simulink model "crop_simulation"  (R2021a)
settings: Solver=ode23tb  StartTime=0.0  StopTime=4  RelTol=1e-2
values from neighbouring files (symbols this model uses):
  parameters = LoadParameters()    [OnlyPlots.m]    (also in run_crop_simulation.m; run_several_crop_simulation.m)
undefined symbols (not defined in the file or in its folder): climate_GH3, MM_vec, nearst_p, p, PowerArtificial, Tr, Tref, Ts, x0_SOFC
libraries: HORTISIM x14, pid_lib x4
(part 1 of 3)
settings Model: SimulationMode=accelerator  Creator=izaro.garro  LastModifiedBy=djoroya
settings SolverCC: AlgebraicLoopSolver=TrustRegion  MinimalZcImpactIntegration=on
settings DebuggingCC: UnconnectedInputMsg=none  UnconnectedOutputMsg=none  UnconnectedLineMsg=none  SFMachineParentedDataDiag=warning
settings SFSimCC: CustomCodeUndefinedFunction=UseInterfaceOnly

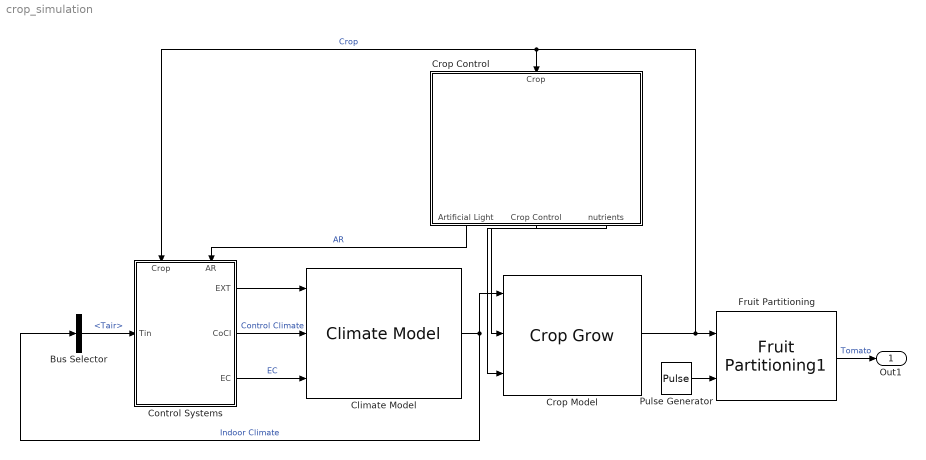
== system crop_simulation ==
  Bus Selector : BusSelector  OutputSignals=Temp.Tair
  Climate Model : HORTISIM/Climate/Models/Climate Model  G0=parameters.climate.G0  T0=parameters.climate.T0  H=parameters.climate.H  A_f=parameters.climate.A_f  A_c=parameters.climate.A_c  minWindows=parameters.climate.minWindows  lam_s=parameters.climate.lam_s  c_s=parameters.climate.c_s  l_s=parameters.climate.l_s  rhod_s=parameters.climate.rhod_s  int_air_speed=parameters.climate.int_air_speed  alpha_i=parameters.climate.alpha_i  alpha_c=parameters.climate.alpha_c  tau_c=parameters.climate.tau_c  alpha_f=parameters.climate.alpha_f  d_c=parameters.climate.d_c  cd_c=parameters.climate.cd_c  T_ss=parameters.climate.T_ss
      settings: SourceProductName=Horti Simulator
  Control Systems : Subsystem
      settings: PortSchema="{\"entries\":[{\"content\":{\"sides\":[{\"content\":{\"connectorIds\":[\"In1\"]},\"type\":\"ConnectorPlacement.EquallySpacedRectSide\",\"uuid\":\"2391a20f-f100-4cab-96a6-b0b26723d027\"},{\"content\":{\"connectorIds\":[\"Out1\",\"Out2\",\"Out3\"],\"side\":\"RIGHT\"},\"type\":\"ConnectorPlacement.EquallySpacedRectSide\",\"uuid\":\"6fe3ba53-dc35-4946-8b7e-8d400e08f612\"},{\"content\":{\"connectorIds\":[\"In2\",\"In3\"],\"side\":\"TOP\"},\"type\":\"ConnectorPlacement.EquallySpacedRectSide\",\"uuid\":\"3c9d9863-f637-4420-aa21-e61bd2fd014c\"}]},\"type\":\"ConnectorPlacement.EquallySpacedConnector\",\"uuid\":\"bf96f136-6ce3-41a6-8557-bc451a3eeee3\"}],\"packageUris\":[\"http://schema.mathworks.com/mf0/Connector/R2020b\"],\"version\":\"1.0\"}"
  Crop Control : Subsystem
  Crop Model : HORTISIM/Horticulture/Models/Crop Grow  Chi_nutrients=parameters.crop.Chi_nutrients  A_v=parameters.crop.A_v  plants_density=parameters.crop.plants_density  fraction_DM=parameters.crop.fraction_DM  min_water_capacity=parameters.crop.min_water_capacity  C_buf_max=parameters.crop.C_buf_max  T_v_start_fruit=parameters.crop.T_v_start_fruit  int_air_speed=parameters.crop.int_air_speed  b_N_uptake=parameters.crop.b_N_uptake  Tv=parameters.crop.Tv  C=parameters.crop.C  R=parameters.crop.R  Tsum=parameters.crop.Tsum  C_wv=parameters.crop.C_wv  N=parameters.crop.N  rg_fruit=parameters.crop.rg_fruit  c_fruit_m=parameters.crop.c_fruit_m  c_fruit_g=parameters.crop.c_fruit_g  rg_leaf=parameters.crop.rg_leaf  c_leaf_m=parameters.crop.c_leaf_m  c_leaf_g=parameters.crop.c_leaf_g  rg_stem=parameters.crop.rg_stem  c_stem_m=parameters.crop.c_stem_m  c_stem_g=parameters.crop.c_stem_g  VelocityAbsortion=parameters.crop.VelocityAbsortion  T_max_v=parameters.crop.T_max_v  s_max_T=parameters.crop.s_max_T  s_min_T=parameters.crop.s_min_T  s_buforg_buf=parameters.crop.s_buforg_buf  T_sum_end=parameters.crop.T_sum_end  T_max_v24=parameters.crop.T_max_v24  T_min_v24=parameters.crop.T_min_v24  s_min_T24=parameters.crop.s_min_T24  s_max_T24=parameters.crop.s_max_T24  T_min_v=parameters.crop.T_min_v
      settings: SourceProductName=Horti Simulator
      mask Display: image('$imagefile'); % Use "Edit Image" on toolstrip to change.
  Fruit Partitioning : HORTISIM/Horticulture/Models/Fruit Partitioning1  Cfruit0=1e-3
      settings: SourceProductName=Horti Simulator
  Pulse Generator : DiscretePulseGenerator  PulseType=Time based  Period=364/parameters.crop.n_seasons  PulseWidth=98
  Out1 : Outport
  wires:
  Climate Model/1 -> Bus Selector/1, Crop Model/1  "Indoor Climate"
  Bus Selector/1 -> Control Systems/1(Tin)  "<Tair>"
  Control Systems/1(EXT) -> Climate Model/1
  Control Systems/2(CoCl) -> Climate Model/2  "Control Climate"
  Control Systems/3(EC) -> Climate Model/3  "EC"
  Crop Model/1 -> Fruit Partitioning/1, Control Systems/2(Crop), Crop Control/1(Crop)  "Crop"
  Crop Control/2("Crop Control ") -> Crop Model/2
  Crop Control/3(nutrients) -> Crop Model/3
  Pulse Generator/1 -> Fruit Partitioning/2
  Fruit Partitioning/1 -> Out1/1  "Tomato"
  Crop Control/1(Artificial Light) -> Control Systems/3(AR)  "AR"

== system crop_simulation/Control Systems ==
  note: Flujo de Calor y Transpiracion
      | desde la planta al aire interior del invernadero
  Tin : Inport
  In Bus Element : Inport  Port=2  PortName=Crop  Element=HeatVars.QT
  In Bus Element1 : Inport  Port=2  PortName=Crop  Element=HeatVars.QV
  In Bus Element2 : Inport  Port=2  PortName=Crop  Element=A_v
  In Bus Element3 : Inport  Port=2  PortName=Crop  Element=CC
  AR : Inport  Port=3
  Heater : Subsystem  Variant=on  VariantControlMode=label  VariantControl=Choice  LabelModeActiveChoice=PID
  "Kelvin2ºC " : HORTISIM/Other  Functions/Kelvin2ºC  SystemSampleTime=-1  VariantActivationTime=update diagram  Latency=0  AutoFrameSizeCalculation=off
      settings: SourceProductName=Horti Simulator
  "Scalar2Bus Ext Signal " : HORTISIM/Other  Functions/Scalar2Bus Ext Signal    SystemSampleTime=-1  VariantActivationTime=update diagram  Latency=0  AutoFrameSizeCalculation=off
      settings: SourceProductName=Horti Simulator
  "Shade Screen and Windows " : Subsystem
  Subsystem4 : Subsystem
  Sum : Sum  Inputs=++|
  EXT : Outport
  CoCl : Outport  Port=2
  EC : Outport  Port=3
  wires:
  Subsystem4/1(EC) -> EC/1
  "Scalar2Bus Ext Signal "/1 -> EXT/1
  AR/1 -> Heater/1(Electrical Power Demand)
  Heater/1(Heater) -> Sum/2  "Potencia calor"
  "Shade Screen and Windows "/1(CoCl) -> CoCl/1
  Tin/1 -> "Kelvin2ºC "/1
  "Kelvin2ºC "/1 -> "Shade Screen and Windows "/1(Ti [ºC]), Heater/2(Ti [ºC])
  In Bus Element/1 -> "Scalar2Bus Ext Signal "/2
  Sum/1 -> "Scalar2Bus Ext Signal "/1
  In Bus Element2/1 -> "Scalar2Bus Ext Signal "/3
  In Bus Element3/1 -> "Scalar2Bus Ext Signal "/4
  In Bus Element1/1 -> Sum/1

== system crop_simulation/Crop Control ==
  Crop : Inport
  From Workspace5 : FromWorkspace  VariableName=Si  ZeroCross=off
  Gain : Gain  Gain=parameters.PowerArtificial
  Gain1 : Gain  Gain=500
  Infinite Water and Nutrients : HORTISIM/Other  Functions/Infinite Water and Nutrients  SystemSampleTime=-1  VariantActivationTime=update diagram  Latency=0  AutoFrameSizeCalculation=off
      settings: SourceProductName=Horti Simulator
  "Lighting System " : Subsystem  Variant=on  VariantControlMode=label  VariantControl=Choice  LabelModeActiveChoice=Choice
  Prune Policy : HORTISIM/Horticulture/Controls/Prune Policy  SystemSampleTime=-1  VariantActivationTime=update diagram  Latency=0  AutoFrameSizeCalculation=off
      settings: SourceProductName=Horti Simulator
  Pulse Generator : DiscretePulseGenerator  PulseType=Time based  Period=364/parameters.crop.n_seasons  PulseWidth=98
  Scalar2Bus Control Crop : HORTISIM/Other  Functions/Scalar2Bus Control Crop  SystemSampleTime=-1  VariantActivationTime=update diagram  Latency=0  AutoFrameSizeCalculation=off
      settings: SourceProductName=Horti Simulator
  Artificial Light : Outport
  "Crop Control " : Outport  Port=2
  nutrients : Outport  Port=3
  wires:
  Pulse Generator/1 -> Scalar2Bus Control Crop/4
  Crop/1 -> Infinite Water and Nutrients/1, Prune Policy/1
  Prune Policy/1 -> Scalar2Bus Control Crop/1
  Infinite Water and Nutrients/1 -> nutrients/1
  Scalar2Bus Control Crop/1 -> "Crop Control "/1
  Gain/1 -> Artificial Light/1
  From Workspace5/1 -> "Lighting System "/1(Si [W/m^2])  "Si"
  "Lighting System "/1(on_off) -> Gain/1  "LightingSystem"
  "Lighting System "/2(AR) -> Gain1/1
  Gain1/1 -> Scalar2Bus Control Crop/3

== system crop_simulation/Control Systems/Heater ==
  Electrical Power Demand : Inport
  Ti [ºC] : Inport  Port=2
  PID : Subsystem  VariantControl=PID
  SOFC : Subsystem  VariantControl=SOFC
  SOFC cascada : Subsystem  VariantControl=SOFC cascada
  Heater : Outport

== system crop_simulation/Control Systems/Shade Screen and Windows  ==
  Ti [ºC] : Inport
  AR [m^2] : Constant  Value=2
  Constant : Constant  Value=0.6
  From Workspace8 : FromWorkspace  VariableName=Si  ZeroCross=off
  Scalar2Bus Control Climate : HORTISIM/Other  Functions/Scalar2Bus  Control Climate  SystemSampleTime=-1  VariantActivationTime=update diagram  Latency=0  AutoFrameSizeCalculation=off
      settings: SourceProductName=Horti Simulator
  Screen : Subsystem
  Screen Connector : HORTISIM/Other  Functions/Screen Connector  SystemSampleTime=-1  VariantActivationTime=update diagram  Latency=0  AutoFrameSizeCalculation=off
      settings: SourceProductName=Horti Simulator
  Windows Connector : HORTISIM/Other  Functions/Windows Connector  SystemSampleTime=-1  VariantActivationTime=update diagram  Latency=0  AutoFrameSizeCalculation=off
      settings: SourceProductName=Horti Simulator
  "Windows " : Subsystem
  CoCl : Outport
  wires:
  From Workspace8/1 -> Screen/1(Rad)
  Windows Connector/1 -> Scalar2Bus Control Climate/1
  Ti [ºC]/1 -> "Windows "/1(Tin)
  Screen/1(Screen) -> Screen Connector/1
  Constant/1 -> Screen Connector/2
  AR [m^2]/1 -> Windows Connector/2
  Scalar2Bus Control Climate/1 -> CoCl/1
  "Windows "/1(Windows) -> Windows Connector/1
  Screen Connector/1 -> Scalar2Bus Control Climate/2

== system crop_simulation/Control Systems/Subsystem4 ==
  Constant : Constant  Value=440
  From Workspace10 : FromWorkspace  VariableName=vv  ZeroCross=off
  From Workspace7 : FromWorkspace  VariableName=tt  ZeroCross=off
  From Workspace8 : FromWorkspace  VariableName=HR  ZeroCross=off
  From Workspace9 : FromWorkspace  VariableName=Si  ZeroCross=off
  Scalar2Bus ExternalClimate : HORTISIM/Other  Functions/Scalar2Bus ExternalClimate  SystemSampleTime=-1  VariantActivationTime=update diagram  Latency=0  AutoFrameSizeCalculation=off
      settings: SourceProductName=Horti Simulator
  Subsystem : Subsystem
  EC : Outport
  wires:
  Scalar2Bus ExternalClimate/1 -> EC/1
  From Workspace8/1 -> Scalar2Bus ExternalClimate/3
  From Workspace10/1 -> Scalar2Bus ExternalClimate/4  "Velocidad viento"
  From Workspace9/1 -> Scalar2Bus ExternalClimate/2
  Constant/1 -> Scalar2Bus ExternalClimate/5
  From Workspace7/1 -> Subsystem/1(In1)
  Subsystem/1(Out1) -> Scalar2Bus ExternalClimate/1

== system crop_simulation/Crop Control/Lighting System  ==
  Si [W/m^2] : Inport
  "Lighting System " : Subsystem  VariantControl=Choice  mask{MinRadAcum=parameters.MAR, MaxDuration=5, RadMaxPower=parameters.PowerArtificial*0.7488}
      mask prompts: MinRadAcum "Minimum Acumulated Radiation (J/m^2)"; MaxDuration "Maximum Duration (hours)"; RadMaxPower "Radiation Power (W)"
  ON : Subsystem  VariantControl=Choice_1
  on_off : Outport
  AR : Outport  Port=2

== system crop_simulation/Control Systems/Heater/PID ==
  Ti [ºC] : Inport
  PID Controller1 : pid_lib/PID Controller  Controller=PID  Form=Parallel  TimeDomain=Continuous-time  UseExternalTs=off  SampleTime=-1  IntegratorMethod=Forward Euler  FilterMethod=Forward Euler  ControllerParametersSource=internal  P=20  I=2*(24*3600)*2/1200  D=0  UseFilter=on  N=0.0006  TunerSelectOption=Transfer Function Based (PID Tuner App)  ZeroCross=off  InitialConditionSource=internal  InitialConditionForIntegrator=0  InitialConditionForFilter=0  DifferentiatorICPrevScaledInput=0  ExternalReset=none  TrackingMode=off  Kt=1  LimitOutput=on  SatLimitsSource=internal  UpperSaturationLimit=100  LowerSaturationLimit=0  LinearizeAsGain=on  AntiWindupMode=clamping  Kb=1  POutMin=[]  POutMax=[]  IOutMin=[]  IOutMax=[]  DOutMin=[]  DOutMax=[]  NOutMin=[]  NOutMax=[]  SumOutMin=[]  SumOutMax=[]  SaturationOutMin=[]  SaturationOutMax=[]  PParamMin=[]  PParamMax=[]  IParamMin=[]  IParamMax=[]  DParamMin=[]  DParamMax=[]  NParamMin=[]  NParamMax=[]  KbParamMin=[]  KbParamMax=[]  KtParamMin=[]  KtParamMax=[]  KbOutMin=[]  KbOutMax=[]  KtOutMin=[]  KtOutMax=[]  IntegratorOutMin=[]  IntegratorOutMax=[]  FilterOutMin=[]  FilterOutMax=[]  SumI1OutMin=[]  SumI1OutMax=[]  SumI2OutMin=[]  SumI2OutMax=[]  SumI3OutMin=[]  SumI3OutMax=[]  SumI4OutMin=[]  SumI4OutMax=[]  SumDOutMin=[]  SumDOutMax=[]  DifferentiatorOutMin=[]  DifferentiatorOutMax=[]  FilterDiffOutCoefMin=[]  FilterDiffOutCoefMax=[]  ReciprocalOutMin=[]  ReciprocalOutMax=[]  SumDenOutMin=[]  SumDenOutMax=[]  SumNumOutMin=[]  SumNumOutMax=[]  DivideOutMin=[]  DivideOutMax=[]  UdiffTsProdOutMin=[]  UdiffTsProdOutMax=[]  NTsProdOutMin=[]  NTsProdOutMax=[]  UintegralTsProdOutMin=[]  UintegralTsProdOutMax=[]  UngainTsProdOutMin=[]  UngainTsProdOutMax=[]  IntegratorContinuousStateAttributes=''  IntegratorStateMustResolveToSignalObject=off  IntegratorRTWStateStorageClass=Auto  FilterContinuousStateAttributes=''  FilterStateMustResolveToSignalObject=off  FilterRTWStateStorageClass=Auto  ParallelPVariant=InternalParameters  IdealPVariant=Disabled  IVariant=InternalParameters  DVariant=InternalParameters  IntegratorVariant=Continuous  SatVariant=Enabled  AWVariant=ContClampingParallel  PCopyVariant=Disabled  TRVariant=Disabled  FdbkBlocksVariant=Forward  IdealPFdbkVariant=Disabled  SatFdbkVariant=Disabled  DerivativeFilterVariant=ContFilter  NVariant=InternalParameters  NCopyVariant=Disabled  FilterICVariant=InternalICsFilter  IntegratorICVariant=InternalICs  ExternalResetVariant=Disabled  TRSumVariant=Passthrough  SumFdbkVariant=Disabled  SumVariant=Sum_PID  TsampFilterVariant=InternalTs  TsampNgainVariant=Passthrough  TsampIntegralVariant=Passthrough  ExternalSaturationOutDataTypeStr=Inherit: Same as second input
  Scope : Scope  NumInputPorts=3
  Sum1 : Sum  Inputs=|+-
  Trefencia1 : Constant  Value=parameters.Tref
  Vector Concatenate : Concatenate
  pila & válvula1 : TransferFcn  Numerator=[6000/(100*1800)]  Denominator=[1/(3600*24) 1/1800]
  Heater : Outport
  wires:
  pila & válvula1/1 -> Scope/1, Heater/1  "Potencia calor"
  Ti [ºC]/1 -> Vector Concatenate/2, Sum1/2
  Trefencia1/1 -> Vector Concatenate/1, Sum1/1
  Sum1/1 -> PID Controller1/1
  PID Controller1/1 -> Scope/3, pila & válvula1/1
  Vector Concatenate/1 -> Scope/2

== system crop_simulation/Control Systems/Heater/SOFC ==
  Electrical Power Demand : Inport
  Ti [ºC] : Inport  Port=2
  Battery : Subsystem
      settings: PortSchema="{\"entries\":[{\"content\":{\"sides\":[{\"content\":{\"connectorIds\":[\"In1\",\"In2\"]},\"type\":\"ConnectorPlacement.EquallySpacedRectSide\",\"uuid\":\"1925230b-a3e9-4566-84e4-810928d751bb\"},{\"content\":{\"connectorIds\":[\"Out1\"],\"side\":\"RIGHT\"},\"type\":\"ConnectorPlacement.EquallySpacedRectSide\",\"uuid\":\"9ffe942e-2098-45f8-a538-edeb3c1d9666\"},{\"content\":{\"connectorIds\":[\"Out2\"],\"side\":\"TOP\"},\"type\":\"ConnectorPlacement.EquallySpacedRectSide\",\"uuid\":\"3c139400-cfdf-443d-b30f-e465049f73b4\"}]},\"type\":\"ConnectorPlacement.EquallySpacedConnector\",\"uuid\":\"3949d6ab-3fdd-4995-b1df-b2b4ee3ea214\"}],\"packageUris\":[\"http://schema.mathworks.com/mf0/Connector/R2020b\"],\"version\":\"1.0\"}"
  Control OP : Subsystem
  Heating Rod : Subsystem
  Kelvin2ºC : HORTISIM/Other  Functions/Kelvin2ºC  SystemSampleTime=-1  VariantActivationTime=update diagram  Latency=0  AutoFrameSizeCalculation=off
      settings: SourceProductName=Horti Simulator
  Reformer  - SOFC System : Subsystem
      settings: PortSchema="{\"entries\":[{\"content\":{\"sides\":[{\"content\":{\"connectorIds\":[\"In1\"]},\"type\":\"ConnectorPlacement.EquallySpacedRectSide\",\"uuid\":\"200e76d3-d0bd-400d-80aa-1287817324e9\"},{\"content\":{\"connectorIds\":[\"Out1\",\"Out2\",\"Out3\"],\"side\":\"RIGHT\"},\"type\":\"ConnectorPlacement.EquallySpacedRectSide\",\"uuid\":\"3a1b6d1c-88bc-44b4-af37-27ac9ade1ff0\"},{\"content\":{\"connectorIds\":[\"In2\",\"In3\",\"In4\"],\"side\":\"TOP\"},\"type\":\"ConnectorPlacement.EquallySpacedRectSide\",\"uuid\":\"7d8c75f4-d537-4a2f-8caa-a1e3e4142219\"},{\"content\":{\"connectorIds\":[],\"side\":\"BOTTOM\"},\"type\":\"ConnectorPlacement.EquallySpacedRectSide\",\"uuid\":\"773ed184-9145-4e58-8690-ed7d817bf4e6\"}]},\"type\":\"ConnectorPlacement.EquallySpacedConnector\",\"uuid\":\"9e56a9e7-d63f-4491-bdfd-789be4cca736\"}],\"packageUris\":[\"http://schema.mathworks.com/mf0/Connector/R2020b\"],\"version\":\"1.0\"}"
  Scope : Scope  NumInputPorts=2
  Scope1 : Scope
  Subsystem2 : Subsystem  Variant=on  VariantControlMode=label  VariantControl=Choice  LabelModeActiveChoice=Choice_1
      settings: PortSchema="{\"entries\":[{\"content\":{\"sides\":[{\"content\":{\"connectorIds\":[]},\"type\":\"ConnectorPlacement.EquallySpacedRectSide\",\"uuid\":\"50e66820-cd92-43dd-993d-153df9ce0354\"},{\"content\":{\"connectorIds\":[\"Out1\"],\"side\":\"RIGHT\"},\"type\":\"ConnectorPlacement.EquallySpacedRectSide\",\"uuid\":\"8d846ca4-6643-48b0-8da4-4b4514e8854e\"},{\"content\":{\"connectorIds\":[],\"side\":\"TOP\"},\"type\":\"ConnectorPlacement.EquallySpacedRectSide\",\"uuid\":\"89928db1-0ab3-4d04-989b-518ec70b2ccf\"},{\"content\":{\"connectorIds\":[\"In1\",\"In2\"],\"side\":\"BOTTOM\"},\"type\":\"ConnectorPlacement.EquallySpacedRectSide\",\"uuid\":\"66b6a137-7b68-4b0a-af93-6c739e693fcb\"}]},\"type\":\"ConnectorPlacement.EquallySpacedConnector\",\"uuid\":\"417f6773-c64e-42aa-b1d6-ce4fc249f7a2\"}],\"packageUris\":[\"http://schema.mathworks.com/mf0/Connector/R2020b\"],\"version\":\"1.0\"}"
  Sum : Sum  Inputs=|++
  Temp. Reformer [K] : Constant  Value=Tr
  Temp. SOFC [K] : Constant  Value=Ts
  "Water Tank " : Subsystem
  Heater : Outport
  wires:
  Temp. SOFC [K]/1 -> Reformer  - SOFC System/4(Ts [K])
  Reformer  - SOFC System/3(Total Power [W]) -> Scope/1
  Temp. Reformer [K]/1 -> Reformer  - SOFC System/3(Tr [K])
  Electrical Power Demand/1 -> Sum/1, Heating Rod/1(" Demand")  "Demand"
  Reformer  - SOFC System/1(Qe [W]) -> Battery/1(Qe [W]), Subsystem2/2(EPD)  "Q SOFC electrical"
  Reformer  - SOFC System/2(Qt [W]) -> "Water Tank "/2(Qt [W])  "Q SOFC thermal"
  Ti [ºC]/1 -> "Water Tank "/1(Ti)
  "Water Tank "/1(Heater) -> Scope1/1, Heater/1
  Control OP/1(OP) -> Reformer  - SOFC System/1(OP)
  "Water Tank "/2(Tw) -> Kelvin2ºC/1, Control OP/1(Tw)  "Tw"
  Sum/1 -> Battery/2(Demand [W])
  Heating Rod/1(Heat) -> Sum/2
  Kelvin2ºC/1 -> Scope/2
  Battery/2(Qe_target) -> Subsystem2/1(Target)
  Subsystem2/1(I [A]) -> Reformer  - SOFC System/2(I [A])

== system crop_simulation/Control Systems/Heater/SOFC cascada ==
  Electrical Power Demand : Inport
  Ti [ºC] : Inport  Port=2
  Battery : Subsystem
      settings: PortSchema="{\"entries\":[{\"content\":{\"sides\":[{\"content\":{\"connectorIds\":[\"In1\"]},\"type\":\"ConnectorPlacement.EquallySpacedRectSide\",\"uuid\":\"0384dfc9-b493-43ca-8976-9edcf8789edb\"},{\"content\":{\"connectorIds\":[\"In2\"],\"side\":\"RIGHT\"},\"type\":\"ConnectorPlacement.EquallySpacedRectSide\",\"uuid\":\"8c1b7a5e-2e19-45da-98e1-e9babae389b5\"},{\"content\":{\"connectorIds\":[],\"side\":\"TOP\"},\"type\":\"ConnectorPlacement.EquallySpacedRectSide\",\"uuid\":\"fdd345dd-528c-4894-b112-922e7101ff3f\"},{\"content\":{\"connectorIds\":[\"Out1\"],\"side\":\"BOTTOM\"},\"type\":\"ConnectorPlacement.EquallySpacedRectSide\",\"uuid\":\"6bdaf1b9-43a5-4c2f-beae-7d98046497e2\"}]},\"type\":\"ConnectorPlacement.EquallySpacedConnector\",\"uuid\":\"8a0122c3-4e9c-4fda-81c5-c11cc8b02729\"}],\"packageUris\":[\"http://schema.mathworks.com/mf0/Connector/R2020b\"],\"version\":\"1.0\"}"
  Control Operations Points : Subsystem
      settings: PortSchema="{\"entries\":[{\"content\":{\"sides\":[{\"content\":{\"connectorIds\":[]},\"type\":\"ConnectorPlacement.EquallySpacedRectSide\",\"uuid\":\"0384dfc9-b493-43ca-8976-9edcf8789edb\"},{\"content\":{\"connectorIds\":[\"Out1\"],\"side\":\"RIGHT\"},\"type\":\"ConnectorPlacement.EquallySpacedRectSide\",\"uuid\":\"8c1b7a5e-2e19-45da-98e1-e9babae389b5\"},{\"content\":{\"connectorIds\":[],\"side\":\"TOP\"},\"type\":\"ConnectorPlacement.EquallySpacedRectSide\",\"uuid\":\"fdd345dd-528c-4894-b112-922e7101ff3f\"},{\"content\":{\"connectorIds\":[\"In1\",\"In2\"],\"side\":\"BOTTOM\"},\"type\":\"ConnectorPlacement.EquallySpacedRectSide\",\"uuid\":\"d5b17d32-762c-4641-a1d6-65705f46c07a\"}]},\"type\":\"ConnectorPlacement.EquallySpacedConnector\",\"uuid\":\"8a0122c3-4e9c-4fda-81c5-c11cc8b02729\"}],\"packageUris\":[\"http://schema.mathworks.com/mf0/Connector/R2020b\"],\"version\":\"1.0\"}"
  Electrical Heating Rod : Subsystem
  Reformer + SOFC : Subsystem
      settings: PortSchema="{\"entries\":[{\"content\":{\"sides\":[{\"content\":{\"connectorIds\":[\"In1\"]},\"type\":\"ConnectorPlacement.EquallySpacedRectSide\",\"uuid\":\"4cd5c40a-1c97-4473-a20a-5da3312550d3\"},{\"content\":{\"connectorIds\":[\"Out1\",\"Out2\"],\"side\":\"RIGHT\"},\"type\":\"ConnectorPlacement.EquallySpacedRectSide\",\"uuid\":\"d0979acb-3e73-453b-a421-f92f187e73e0\"},{\"content\":{\"connectorIds\":[\"In2\"],\"side\":\"TOP\"},\"type\":\"ConnectorPlacement.EquallySpacedRectSide\",\"uuid\":\"eaeaf2a9-9974-4812-b222-1ca0797dcdde\"}]},\"type\":\"ConnectorPlacement.EquallySpacedConnector\",\"uuid\":\"9fd2fb58-b934-4df9-8ab3-03deaf4be922\"}],\"packageUris\":[\"http://schema.mathworks.com/mf0/Connector/R2020b\"],\"version\":\"1.0\"}"
  Sum : Sum  Inputs=|++
  "Water Tank " : Subsystem
      settings: PortSchema="{\"entries\":[{\"content\":{\"sides\":[{\"content\":{\"connectorIds\":[\"In1\"]},\"type\":\"ConnectorPlacement.EquallySpacedRectSide\",\"uuid\":\"d29156f9-e2c2-4586-825a-d86d133af181\"},{\"content\":{\"connectorIds\":[\"Out1\"],\"side\":\"RIGHT\"},\"type\":\"ConnectorPlacement.EquallySpacedRectSide\",\"uuid\":\"4d2f4769-faea-4a23-a13d-339e92b1d630\"},{\"content\":{\"connectorIds\":[\"In2\"],\"side\":\"TOP\"},\"type\":\"ConnectorPlacement.EquallySpacedRectSide\",\"uuid\":\"30773c19-fd81-4dd5-9729-b7dacfd09c59\"},{\"content\":{\"connectorIds\":[\"Out2\",\"In3\"],\"side\":\"BOTTOM\"},\"type\":\"ConnectorPlacement.EquallySpacedRectSide\",\"uuid\":\"b58df793-d7ca-48f5-b5d9-4f9f6338e59f\"}]},\"type\":\"ConnectorPlacement.EquallySpacedConnector\",\"uuid\":\"dfac1afe-3db7-49cf-a21d-7cea522fc355\"}],\"packageUris\":[\"http://schema.mathworks.com/mf0/Connector/R2020b\"],\"version\":\"1.0\"}"
  Heater : Outport
  wires:
  "Water Tank "/1(Heater [W]) -> Heater/1
  "Water Tank "/2(Tw [K]) -> Control Operations Points/2(Tw [K])  "Tw"
  Electrical Heating Rod/1(Heat) -> "Water Tank "/2(Rod), Sum/2
  Electrical Power Demand/1 -> Sum/1, Electrical Heating Rod/1(" Demand")  "Artificial Lighting  Demand"
  Ti [ºC]/1 -> Control Operations Points/1(Ti [ºC]), "Water Tank "/3(Ti [ºC])
  Sum/1 -> Battery/1(TED [W])  "Total  Electrical  Demand"
  Battery/1(I [A]) -> Reformer + SOFC/2(I [A])
  Control Operations Points/1(OP) -> Reformer + SOFC/1(OP)
  Reformer + SOFC/1(Q SOFC e) -> Battery/2(QSOFC_e [W])
  Reformer + SOFC/2(Q SOFC th) -> "Water Tank "/1(QSOCF [W])

== system crop_simulation/Control Systems/Shade Screen and Windows /Screen ==
  Rad : Inport
  If : If  IfExpression=u1 < 15
  If Action Subsystem : Subsystem  TreatAsAtomicUnit=on
  If Action Subsystem1 : Subsystem  TreatAsAtomicUnit=on
  Merge : Merge
  Screen : Outport
  wires:
  Rad/1 -> If Action Subsystem1/1(in), If/1
  Merge/1 -> Screen/1
  If/1 -> If Action Subsystem/Action
  If/2 -> If Action Subsystem1/Action
  If Action Subsystem/1(Out1) -> Merge/1
  If Action Subsystem1/1(Out1) -> Merge/2

== system crop_simulation/Control Systems/Shade Screen and Windows /Windows  ==
  Tin : Inport
  Constant : Constant  Value=20
  Gain : Gain  Gain=0.5
  Gain1 : Gain  Gain=100
  Minus : Sum  Inputs=-+
  Saturation : Saturate  UpperLimit=1  LowerLimit=0  ZeroCross=off
  Windows : Outport
  wires:
  Tin/1 -> Minus/2
  Constant/1 -> Minus/1
  Minus/1 -> Gain/1
  Gain/1 -> Saturation/1
  Saturation/1 -> Gain1/1
  Gain1/1 -> Windows/1

== system crop_simulation/Control Systems/Subsystem4/Subsystem ==
  In1 : Inport
  Constant : Constant  Value=273.15
  Sum : Sum  Inputs=|++
  Out1 : Outport
  wires:
  Sum/1 -> Out1/1
  In1/1 -> Sum/1
  Constant/1 -> Sum/2

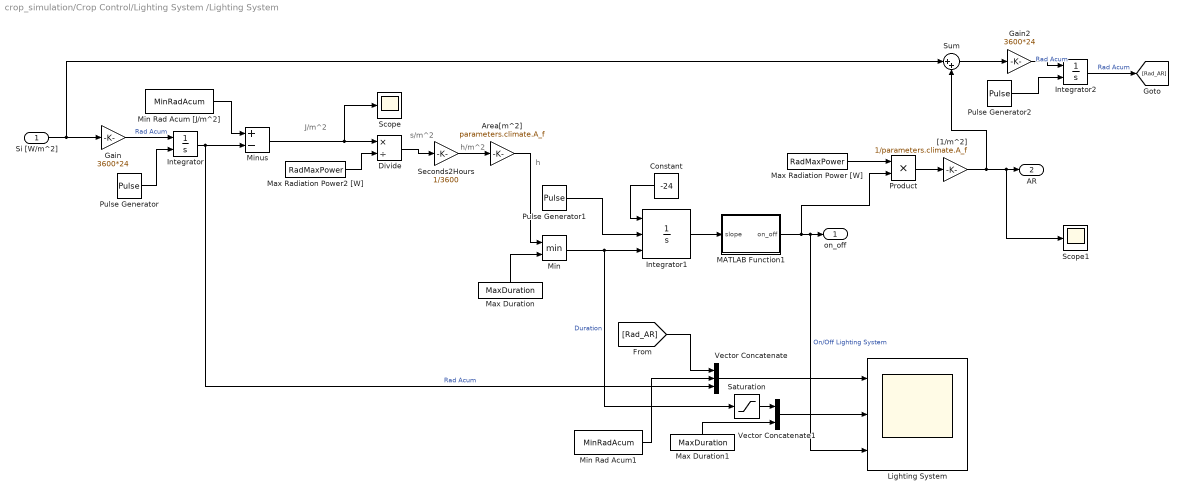
== system crop_simulation/Crop Control/Lighting System /Lighting System  ==
  note: J/m^2
  note: s/m^2
  note: h/m^2
  note: h
  Si [W/m^2] : Inport
  Area[m^2] : Gain  Gain=parameters.climate.A_f
  Constant : Constant  Value=-24
  Divide : Product  Inputs=*/
  Gain : Gain  Gain=3600*24
  Gain2 : Gain  Gain=3600*24
  Integrator : Integrator  ExternalReset=rising
  Integrator1 : Integrator  ExternalReset=rising  InitialConditionSource=external
  Integrator2 : Integrator  ExternalReset=rising
  Lighting System : Scope  NumInputPorts=3
  MATLAB Function1 : MATLAB Function  TreatAsAtomicUnit=on
  Max Duration : Constant  Value=MaxDuration
  Max Duration1 : Constant  Value=MaxDuration
  Max Radiation Power [W] : Constant  Value=RadMaxPower
  Max Radiation Power2 [W] : Constant  Value=RadMaxPower
  Min : MinMax  Inputs=2  ZeroCross=off
  Min Rad Acum [J/m^2] : Constant  Value=MinRadAcum
  Min Rad Acum1 : Constant  Value=MinRadAcum
  Minus : Sum  Inputs=+-
  Product : Product
  Pulse Generator : DiscretePulseGenerator  PulseType=Time based  Period=1  PulseWidth=5  PhaseDelay=0.05
  Pulse Generator1 : DiscretePulseGenerator  PulseType=Time based  Period=1  PulseWidth=5  PhaseDelay=22/24
  Pulse Generator2 : DiscretePulseGenerator  PulseType=Time based  Period=1  PulseWidth=5  PhaseDelay=0.05
  Saturation : Saturate  UpperLimit=inf  LowerLimit=0
  Scope : Scope
  Scope1 : Scope
  Seconds2Hours : Gain  Gain=1/3600
  Sum : Sum  Inputs=|++
  Vector Concatenate : Concatenate  NumInputs=3
  Vector Concatenate1 : Concatenate
  "[1/m^2]" : Gain  Gain=1/parameters.climate.A_f
  on_off : Outport
  AR : Outport  Port=2
  wires:
  MATLAB Function1/1(on_off) -> on_off/1, Lighting System/3, Product/2  "On/Off Lighting System"
  Integrator1/1 -> MATLAB Function1/1(slope)
  Pulse Generator/1 -> Integrator/2
  Constant/1 -> Integrator1/1
  Integrator/1 -> Minus/2, Vector Concatenate/3  "Rad Acum"
  Vector Concatenate/1 -> Lighting System/1
  Min/1 -> Saturation/1, Integrator1/3  "Duration"
  Max Radiation Power [W]/1 -> Product/1
  Product/1 -> "[1/m^2]"/1
  "[1/m^2]"/1 -> Scope1/1, AR/1, Sum/2
  Pulse Generator1/1 -> Integrator1/2
  Max Duration/1 -> Min/2
  Min Rad Acum1/1 -> Vector Concatenate/2
  Vector Concatenate1/1 -> Lighting System/2
  Max Duration1/1 -> Vector Concatenate1/2
  Divide/1 -> Seconds2Hours/1
  Minus/1 -> Scope/1, Divide/1
  Min Rad Acum [J/m^2]/1 -> Minus/1
  Max Radiation Power2 [W]/1 -> Divide/2
  Si [W/m^2]/1 -> Gain/1, Sum/1
  Gain/1 -> Integrator/1  "Rad Acum"
  Pulse Generator2/1 -> Integrator2/2
  Sum/1 -> Gain2/1
  Gain2/1 -> Integrator2/1  "Rad Acum"
  Integrator2/1 -> [Rad_AR]  "Rad Acum"
  [Rad_AR] -> Vector Concatenate/1
  Seconds2Hours/1 -> Area[m^2]/1
  Area[m^2]/1 -> Min/1
  Saturation/1 -> Vector Concatenate1/1

== system crop_simulation/Crop Control/Lighting System /ON ==
  Constant : Constant
  Constant1 : Constant  Value=PowerArtificial * 0.7488
  Gain1 : Gain  Gain=1/climate_GH3.A_f
  Product : Product
  on_off : Outport
  AR : Outport  Port=2
  wires:
  Constant1/1 -> Product/1
  Gain1/1 -> AR/1
  Product/1 -> Gain1/1
  Constant/1 -> Product/2, on_off/1  "On/Off Lighting System"

== system crop_simulation/Control Systems/Heater/SOFC/Battery ==
  Qe [W] : Inport
  Demand [W] : Inport  Port=2
  Constant : Constant  Value=2.84*1000*3600
  Divide : Product  Inputs=*/
  Gain : Gain  Gain=24*3600
  Integrator : Integrator  InitialCondition=2.84*1000*3600/2
  Minus : Sum  Inputs=+-
  Relay : Relay  OnSwitchValue=0.8  OffSwitchValue=0.4  OnOutputValue=0  OffOutputValue=500  ZeroCross=off
  Scope : Scope
  Scope1 : Scope  NumInputPorts=2
  Scope2 : Scope
  SOC : Outport
  Qe_target : Outport  Port=2
  wires:
  Qe [W]/1 -> Minus/1
  Integrator/1 -> Divide/1
  Demand [W]/1 -> Minus/2, Scope2/1
  Relay/1 -> Scope1/1, Qe_target/1
  Constant/1 -> Divide/2
  Divide/1 -> Scope1/2, Scope/1, SOC/1, Relay/1
  Gain/1 -> Integrator/1
  Minus/1 -> Gain/1

== system crop_simulation/Control Systems/Heater/SOFC/Control OP ==
  Tw : Inport
  Constant : Constant  Value=273.15
  Minus : Sum  Inputs=+-
  Select Operation Point : Subsystem  Variant=on  VariantControlMode=label  VariantControl=Choice  LabelModeActiveChoice=Choice_2
  Transformacion Flujos : Subsystem
  OP : Outport
  wires:
  Transformacion Flujos/1(OP) -> OP/1
  Tw/1 -> Minus/1
  Constant/1 -> Minus/2
  Minus/1 -> Select Operation Point/1(Tw [ºC])
  Select Operation Point/1(OP) -> Transformacion Flujos/1(In1)  "OP"

== system crop_simulation/Control Systems/Heater/SOFC/Heating Rod ==
  " Demand" : Inport
  If : If  IfExpression=u1 < 1  ZeroCross=off
  If Action Subsystem : Subsystem  TreatAsAtomicUnit=on
  If Action Subsystem1 : Subsystem  TreatAsAtomicUnit=on
  Merge : Merge
  Heat : Outport
  wires:
  " Demand"/1 -> If/1
  If/1 -> If Action Subsystem/Action
  If/2 -> If Action Subsystem1/Action
  If Action Subsystem/1(Out1) -> Merge/1
  If Action Subsystem1/1(Out1) -> Merge/2
  Merge/1 -> Heat/1

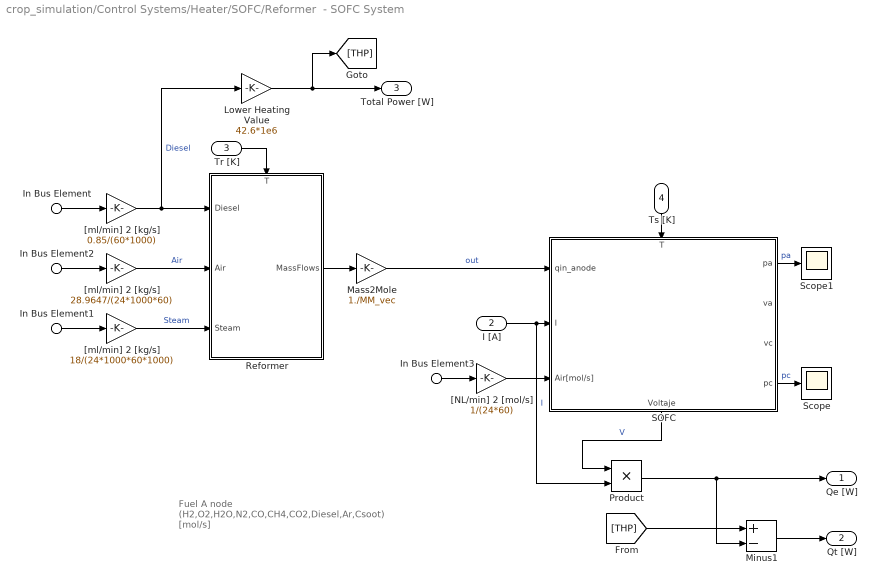
== system crop_simulation/Control Systems/Heater/SOFC/Reformer  - SOFC System ==
  note: Fuel
      | A node
      | (H2,O2,H2O,N2,CO,CH4,CO2,Diesel,Ar,Csoot)
      | [mol/s]
  In Bus Element : Inport  PortName=OP  Element=Diesel [ml/min]
  In Bus Element1 : Inport  PortName=OP  Element=Steam [ml/min]
  In Bus Element2 : Inport  PortName=OP  Element=Air [NL/min]
  In Bus Element3 : Inport  PortName=OP  Element=Air_cath [NL/min]
  I [A] : Inport  Port=2
  Tr [K] : Inport  Port=3
  Ts [K] : Inport  Port=4
  Lower Heating Value : Gain  Gain=42.6*1e6
  Mass2Mole : Gain  Gain=1./MM_vec
  Minus1 : Sum  Inputs=+-
  Product : Product
  "Reformer " : Subsystem
      settings: PortSchema="{\"entries\":[{\"content\":{\"sides\":[{\"content\":{\"connectorIds\":[\"In1\",\"In2\",\"In3\"]},\"type\":\"ConnectorPlacement.EquallySpacedRectSide\",\"uuid\":\"bf799419-3c51-4e41-80c3-8f053955be8d\"},{\"content\":{\"connectorIds\":[\"Out1\"],\"side\":\"RIGHT\"},\"type\":\"ConnectorPlacement.EquallySpacedRectSide\",\"uuid\":\"8203b5dc-5749-4c6f-8169-46d2df527b78\"},{\"content\":{\"connectorIds\":[\"In4\"],\"side\":\"TOP\"},\"type\":\"ConnectorPlacement.EquallySpacedRectSide\",\"uuid\":\"29bf5c31-2b54-418d-a6d2-10fc76893a8c\"}]},\"type\":\"ConnectorPlacement.EquallySpacedConnector\",\"uuid\":\"ce77c350-1f9b-4f0b-aae0-5de0ba71c7e8\"}],\"packageUris\":[\"http://schema.mathworks.com/mf0/Connector/R2020b\"],\"version\":\"1.0\"}"
  "SOFC " : Subsystem  mask{p=p, x0=x0_SOFC}
      mask prompts: p "params"
      settings: PortSchema="{\"entries\":[{\"content\":{\"sides\":[{\"content\":{\"connectorIds\":[\"In1\",\"In2\",\"In3\"]},\"type\":\"ConnectorPlacement.EquallySpacedRectSide\",\"uuid\":\"6cca8e4f-6db2-48de-a60a-b6fbc16877c6\"},{\"content\":{\"connectorIds\":[\"Out1\",\"Out2\",\"Out3\",\"Out4\"],\"side\":\"RIGHT\"},\"type\":\"ConnectorPlacement.EquallySpacedRectSide\",\"uuid\":\"c481f6d1-531d-4215-9ae0-5807376c0625\"},{\"content\":{\"connectorIds\":[\"In4\"],\"side\":\"TOP\"},\"type\":\"ConnectorPlacement.EquallySpacedRectSide\",\"uuid\":\"76720726-927e-4340-b17d-e33f4db2c782\"},{\"content\":{\"connectorIds\":[\"Out5\"],\"side\":\"BOTTOM\"},\"type\":\"ConnectorPlacement.EquallySpacedRectSide\",\"uuid\":\"7ed108e3-6588-44d6-8f3d-9789ffe258a7\"}]},\"type\":\"ConnectorPlacement.EquallySpacedConnector\",\"uuid\":\"f9228f26-0840-43d6-932a-2fdb8a27bf20\"}],\"packageUris\":[\"http://schema.mathworks.com/mf0/Connector/R2020b\"],\"version\":\"1.0\"}"
  Scope : Scope
  Scope1 : Scope
  "[NL/min] 2 [mol/s]" : Gain  Gain=1/(24*60)
  "[ml/min] 2 [kg/s]" : Gain  Gain=0.85/(60*1000)
  "[ml/min] 2 [kg/s] " : Gain  Gain=28.9647/(24*1000*60)
  "[ml/min] 2 [kg/s]  " : Gain  Gain=18/(24*1000*60*1000)
  Qe [W] : Outport
  Qt [W] : Outport  Port=2
  Total Power [W] : Outport  Port=3
  wires:
  I [A]/1 -> "SOFC "/2(I), Product/2  "I"
  "SOFC "/5(Voltaje) -> Product/1  "V"
  Ts [K]/1 -> "SOFC "/4(T)
  Product/1 -> Qe [W]/1, Minus1/2
  In Bus Element/1 -> "[ml/min] 2 [kg/s]"/1
  In Bus Element2/1 -> "[ml/min] 2 [kg/s] "/1
  In Bus Element1/1 -> "[ml/min] 2 [kg/s]  "/1
  In Bus Element3/1 -> "[NL/min] 2 [mol/s]"/1
  "[NL/min] 2 [mol/s]"/1 -> "SOFC "/3(Air[mol/s])
  Lower Heating Value/1 -> Total Power [W]/1, [THP]
  [THP] -> Minus1/1
  Minus1/1 -> Qt [W]/1
  "SOFC "/4(pc) -> Scope/1  "pc"
  "SOFC "/1(pa) -> Scope1/1  "pa"
  "Reformer "/1(MassFlows) -> Mass2Mole/1
  Tr [K]/1 -> "Reformer "/4(T)
  "[ml/min] 2 [kg/s]"/1 -> Lower Heating Value/1, "Reformer "/1(Diesel)  "Diesel"
  "[ml/min] 2 [kg/s] "/1 -> "Reformer "/2(Air)  "Air"
  "[ml/min] 2 [kg/s]  "/1 -> "Reformer "/3(Steam)  "Steam"
  Mass2Mole/1 -> "SOFC "/1(qin_anode)  "out"

== system crop_simulation/Control Systems/Heater/SOFC/Subsystem2 ==
  Target : Inport
  EPD : Inport  Port=2
  Continous : Subsystem  VariantControl=Choice_1
  Subsystem2 : Subsystem  VariantControl=Choice
      settings: PortSchema="{\"entries\":[{\"content\":{\"sides\":[{\"content\":{\"connectorIds\":[]},\"type\":\"ConnectorPlacement.EquallySpacedRectSide\",\"uuid\":\"50e66820-cd92-43dd-993d-153df9ce0354\"},{\"content\":{\"connectorIds\":[],\"side\":\"RIGHT\"},\"type\":\"ConnectorPlacement.EquallySpacedRectSide\",\"uuid\":\"8d846ca4-6643-48b0-8da4-4b4514e8854e\"},{\"content\":{\"connectorIds\":[\"Out1\"],\"side\":\"TOP\"},\"type\":\"ConnectorPlacement.EquallySpacedRectSide\",\"uuid\":\"89928db1-0ab3-4d04-989b-518ec70b2ccf\"},{\"content\":{\"connectorIds\":[\"In1\",\"In2\"],\"side\":\"BOTTOM\"},\"type\":\"ConnectorPlacement.EquallySpacedRectSide\",\"uuid\":\"be94ecfa-8f34-4f3e-bda2-4dff795f79cd\"}]},\"type\":\"ConnectorPlacement.EquallySpacedConnector\",\"uuid\":\"417f6773-c64e-42aa-b1d6-ce4fc249f7a2\"}],\"packageUris\":[\"http://schema.mathworks.com/mf0/Connector/R2020b\"],\"version\":\"1.0\"}"
  I [A] : Outport

== system crop_simulation/Control Systems/Heater/SOFC/Water Tank  ==
  Ti : Inport
  Qt [W] : Inport  Port=2
  Control Law : Subsystem
  Gain : Gain  Gain=24*3600
  Gain2 : Gain  Gain=-1
  Gain3 : Gain  Gain=1/(260*4186)
  Integrator : Integrator  InitialCondition=climate_GH3.T0(2)
  Kelvin2ºC : HORTISIM/Other  Functions/Kelvin2ºC  SystemSampleTime=-1  VariantActivationTime=update diagram  Latency=0  AutoFrameSizeCalculation=off
      settings: SourceProductName=Horti Simulator
  Scope : Scope  NumInputPorts=2
  Sum : Sum  Inputs=+++
  recooling : Subsystem
  Heater : Outport
  Tw : Outport  Port=2
  wires:
  Integrator/1 -> Tw/1, [Tw]
  Gain/1 -> Integrator/1
  [Tw] -> recooling/1(Tw)
  recooling/1(Qrecold) -> Sum/1
  Gain2/1 -> Heater/1
  Sum/1 -> Gain3/1
  Gain3/1 -> Gain/1
  [Tw] -> Control Law/2(Tw)
  Control Law/1(Heat[W]) -> Gain2/1, Sum/3
  Qt [W]/1 -> Sum/2
  [Tw] -> Kelvin2ºC/1
  Kelvin2ºC/1 -> Scope/2
  Ti/1 -> [Ti]
  [Ti] -> Control Law/1(Ti)
  [Ti] -> Scope/1

== system crop_simulation/Control Systems/Heater/SOFC cascada/Battery ==
  note: Battery
  note: Total
      | Electrical
      | Demand
  note: Emulador de
      | Intensidad Electrica a
      | través del
      | (inversor/convertidor de voltaje),
      | con el fin de evitar bucles algebraicos. Dado una demanda electrica se calcula la intensidad que debería atravezar la pila de combustible para producir esa energía electrica
  note: Emulador de
      | Intensidad Electrica a
      | través del
      | (inversor/convertidor de voltaje),
      | con el fin de evitar bucles algebraicos.
      |
      | Se calcula la demanda de potencia electrica que pide la bateria
  note: Potencia Electrica para cargar la bateria. Energia Electrica desde el sistema SOFC, hacia la bateria
  note: Potencia Electrica consumida de la bateria. Esta término es la demanda electrica: Luz artifical y Electrical Heating Rod
  TED [W] : Inport
  QSOFC_e [W] : Inport  Port=2
  Calculo de Corriente atraves de la celda de combustible : Subsystem  Variant=on  VariantControlMode=label  VariantControl=Choice  LabelModeActiveChoice=Choice_1
      settings: PortSchema="{\"entries\":[{\"content\":{\"sides\":[{\"content\":{\"connectorIds\":[]},\"type\":\"ConnectorPlacement.EquallySpacedRectSide\",\"uuid\":\"50e66820-cd92-43dd-993d-153df9ce0354\"},{\"content\":{\"connectorIds\":[],\"side\":\"RIGHT\"},\"type\":\"ConnectorPlacement.EquallySpacedRectSide\",\"uuid\":\"8d846ca4-6643-48b0-8da4-4b4514e8854e\"},{\"content\":{\"connectorIds\":[\"Out1\"],\"side\":\"TOP\"},\"type\":\"ConnectorPlacement.EquallySpacedRectSide\",\"uuid\":\"89928db1-0ab3-4d04-989b-518ec70b2ccf\"},{\"content\":{\"connectorIds\":[\"In1\",\"In2\"],\"side\":\"BOTTOM\"},\"type\":\"ConnectorPlacement.EquallySpacedRectSide\",\"uuid\":\"66b6a137-7b68-4b0a-af93-6c739e693fcb\"}]},\"type\":\"ConnectorPlacement.EquallySpacedConnector\",\"uuid\":\"417f6773-c64e-42aa-b1d6-ce4fc249f7a2\"}],\"packageUris\":[\"http://schema.mathworks.com/mf0/Connector/R2020b\"],\"version\":\"1.0\"}"
  Constant : Constant  Value=2.84*1000*3600
  Control de Carga : Relay  OnSwitchValue=0.8  OffSwitchValue=0.4  OnOutputValue=0  OffOutputValue=500  ZeroCross=off
  Divide : Product  Inputs=*/
  Gain : Gain  Gain=24*3600
  Integrator : Integrator  InitialCondition=2.84*1000*3600/2
  Minus : Sum  Inputs=+-
  I [A] : Outport
  wires:
  Calculo de Corriente atraves de la celda de combustible/1(I [A]) -> I [A]/1
  Divide/1 -> Control de Carga/1  "State  Of  Charge [0-1]"
  Control de Carga/1 -> Calculo de Corriente atraves de la celda de combustible/1(Target)  "Power  Demanded  to charge"
  Minus/1 -> Gain/1
  Gain/1 -> Integrator/1
  Constant/1 -> Divide/2
  TED [W]/1 -> Minus/2
  Integrator/1 -> Divide/1
  QSOFC_e [W]/1 -> Calculo de Corriente atraves de la celda de combustible/2(EPD), Minus/1

== system crop_simulation/Control Systems/Heater/SOFC cascada/Control Operations Points ==
  Ti [ºC] : Inport
  Tw [K] : Inport  Port=2
  Control OP : Subsystem
  Control Tw : Subsystem
  OP : Outport
  wires:
  Ti [ºC]/1 -> Control Tw/1(Ti [ºC])
  Tw [K]/1 -> Control OP/2(Tw [K])
  Control OP/1(OP) -> OP/1
  Control Tw/1(Tw_target [K]) -> Control OP/1(Tw_target [K])

== system crop_simulation/Control Systems/Heater/SOFC cascada/Electrical Heating Rod ==
  " Demand" : Inport
  If : If  IfExpression=u1 < 1  ZeroCross=off
  If Action Subsystem : Subsystem  TreatAsAtomicUnit=on
  If Action Subsystem1 : Subsystem  TreatAsAtomicUnit=on
  Merge : Merge
  Heat : Outport
  wires:
  " Demand"/1 -> If/1
  If/1 -> If Action Subsystem/Action
  If/2 -> If Action Subsystem1/Action
  If Action Subsystem/1(Out1) -> Merge/1
  If Action Subsystem1/1(Out1) -> Merge/2
  Merge/1 -> Heat/1

== system crop_simulation/Control Systems/Heater/SOFC cascada/Reformer + SOFC ==
  OP : Inport
  I [A] : Inport  Port=2
  Reformer  - SOFC System : Subsystem
      settings: PortSchema="{\"entries\":[{\"content\":{\"sides\":[{\"content\":{\"connectorIds\":[\"In1\"]},\"type\":\"ConnectorPlacement.EquallySpacedRectSide\",\"uuid\":\"200e76d3-d0bd-400d-80aa-1287817324e9\"},{\"content\":{\"connectorIds\":[\"Out1\",\"Out2\"],\"side\":\"RIGHT\"},\"type\":\"ConnectorPlacement.EquallySpacedRectSide\",\"uuid\":\"3a1b6d1c-88bc-44b4-af37-27ac9ade1ff0\"},{\"content\":{\"connectorIds\":[\"In2\",\"In3\",\"In4\"],\"side\":\"TOP\"},\"type\":\"ConnectorPlacement.EquallySpacedRectSide\",\"uuid\":\"7d8c75f4-d537-4a2f-8caa-a1e3e4142219\"},{\"content\":{\"connectorIds\":[],\"side\":\"BOTTOM\"},\"type\":\"ConnectorPlacement.EquallySpacedRectSide\",\"uuid\":\"773ed184-9145-4e58-8690-ed7d817bf4e6\"}]},\"type\":\"ConnectorPlacement.EquallySpacedConnector\",\"uuid\":\"9e56a9e7-d63f-4491-bdfd-789be4cca736\"}],\"packageUris\":[\"http://schema.mathworks.com/mf0/Connector/R2020b\"],\"version\":\"1.0\"}"
  Temp. Reformer [K] : Constant  Value=parameters.Heating.Reformer.T
  Temp. SOFC [K] : Constant  Value=parameters.Heating.SOFC.T
  Q SOFC e : Outport
  Q SOFC th : Outport  Port=2
  wires:
  Reformer  - SOFC System/2(Qt [W]) -> Q SOFC th/1  "Q SOFC thermal"
  I [A]/1 -> Reformer  - SOFC System/4(I [A])
  Reformer  - SOFC System/1(Qe [W]) -> Q SOFC e/1  "Q SOFC electrical"
  OP/1 -> Reformer  - SOFC System/1(OP)
  Temp. Reformer [K]/1 -> Reformer  - SOFC System/2(Tr [K])
  Temp. SOFC [K]/1 -> Reformer  - SOFC System/3(Ts [K])

== system crop_simulation/Control Systems/Heater/SOFC cascada/Water Tank  ==
  QSOCF [W] : Inport
  Rod : Inport  Port=2
  Ti [ºC] : Inport  Port=3
  Control Law : Subsystem
  Gain : Gain  Gain=24*3600
  Gain2 : Gain  Gain=-1
  Gain3 : Gain  Gain=1/(260*4186)
  Integrator : Integrator  InitialCondition=70 + 273.15
  Sum : Sum  Inputs=++++
  recooling : Subsystem
  Heater [W] : Outport
  Tw [K] : Outport  Port=2
  wires:
  Integrator/1 -> Tw [K]/1, [Tw]
  Gain/1 -> Integrator/1
  [Tw] -> recooling/1(Tw)
  recooling/1(Qrecold) -> Sum/1
  Gain2/1 -> Heater [W]/1
  Sum/1 -> Gain3/1
  Gain3/1 -> Gain/1
  [Tw] -> Control Law/2(Tw)
  Control Law/1(Heat[W]) -> Gain2/1, Sum/3
  QSOCF [W]/1 -> Sum/2
  Ti [ºC]/1 -> [Ti]
  [Ti] -> Control Law/1(Ti)
  Rod/1 -> Sum/4

== system crop_simulation/Control Systems/Shade Screen and Windows /Screen/If Action Subsystem ==
  Action Port : ActionPort  ActionPortLabel=if(u1 < 15)
  Constant : Constant  Value=0
  Out1 : Outport
  wires:
  Constant/1 -> Out1/1

== system crop_simulation/Control Systems/Shade Screen and Windows /Screen/If Action Subsystem1 ==
  in : Inport
  Action Port : ActionPort  ActionPortLabel=else
  Relay : Relay  OnSwitchValue=300  OffSwitchValue=250  OnOutputValue=100
  Out1 : Outport
  wires:
  in/1 -> Relay/1
  Relay/1 -> Out1/1

== system crop_simulation/Control Systems/Heater/SOFC/Control OP/Select Operation Point ==
  Tw [ºC] : Inport
  Relay : Subsystem  VariantControl=Choice_1
  Relay 3 : Subsystem  VariantControl=Choice_2
  Select Operation Point : Subsystem  VariantControl=Choice
  OP : Outport

== system crop_simulation/Control Systems/Heater/SOFC/Control OP/Transformacion Flujos ==
  In1 : Inport
  If Action Subsystem : Subsystem  TreatAsAtomicUnit=on
  If Action Subsystem1 : Subsystem  TreatAsAtomicUnit=on
  If Action Subsystem2 : Subsystem  TreatAsAtomicUnit=on
  If Action Subsystem3 : Subsystem  TreatAsAtomicUnit=on
  Merge : Merge  Inputs=4
  Rate Limiter : RateLimiter  RisingSlewLimit=500  FallingSlewLimit=-500  SampleTimeMode=inherited
  Scope : Scope  NumInputPorts=2
  Switch Case : SwitchCase  CaseConditions={4,3,2,1}  ShowDefaultCase=off
  OP : Outport
  wires:
  In1/1 -> Switch Case/1
  Switch Case/3 -> If Action Subsystem2/Action
  If Action Subsystem1/1(Out1) -> Merge/2
  If Action Subsystem/1(Out1) -> Merge/1
  If Action Subsystem2/1(Out1) -> Merge/3
  Merge/1 -> Scope/2, Rate Limiter/1, OP/1
  Switch Case/2 -> If Action Subsystem1/Action
  Switch Case/1 -> If Action Subsystem/Action
  Switch Case/4 -> If Action Subsystem3/Action
  If Action Subsystem3/1(Out1) -> Merge/4
  Rate Limiter/1 -> Scope/1

== system crop_simulation/Control Systems/Heater/SOFC/Heating Rod/If Action Subsystem ==
  Action Port : ActionPort  ActionPortLabel=if(u1 < 1)
  Constant : Constant  Value=200
  Out1 : Outport
  wires:
  Constant/1 -> Out1/1

== system crop_simulation/Control Systems/Heater/SOFC/Heating Rod/If Action Subsystem1 ==
  Action Port : ActionPort  ActionPortLabel=else
  Constant : Constant  Value=0
  Out1 : Outport
  wires:
  Constant/1 -> Out1/1

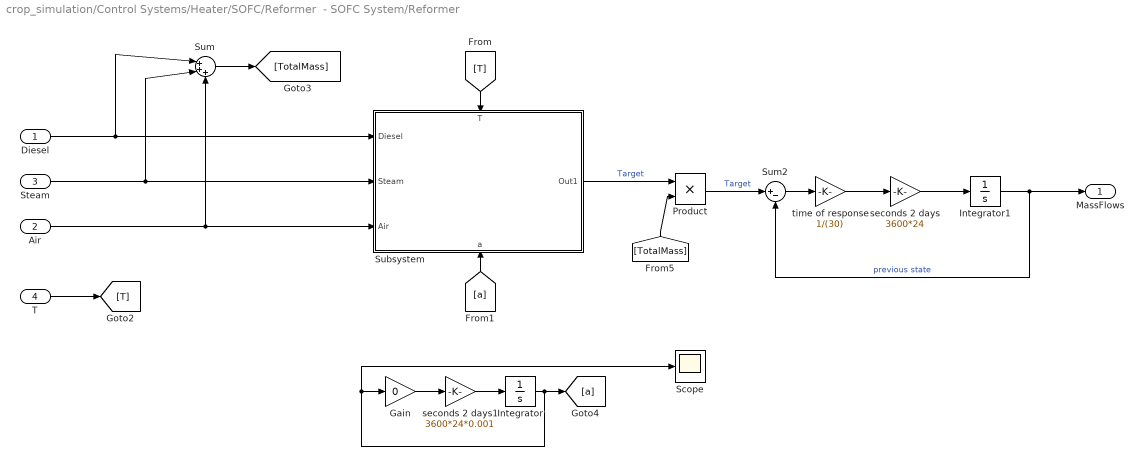
== system crop_simulation/Control Systems/Heater/SOFC/Reformer  - SOFC System/Reformer  ==
  Diesel : Inport
  Air : Inport  Port=2
  Steam : Inport  Port=3
  T : Inport  Port=4
  Gain : Gain  Gain=0
  Integrator : Integrator  InitialCondition=1
  Integrator1 : Integrator  InitialCondition=1e-6
  Product : Product
  Scope : Scope
  Subsystem : Subsystem
      settings: PortSchema="{\"entries\":[{\"content\":{\"sides\":[{\"content\":{\"connectorIds\":[\"In1\",\"In2\",\"In3\"]},\"type\":\"ConnectorPlacement.EquallySpacedRectSide\",\"uuid\":\"0dada652-6957-4c3e-8e48-73ee360a3bab\"},{\"content\":{\"connectorIds\":[\"Out1\"],\"side\":\"RIGHT\"},\"type\":\"ConnectorPlacement.EquallySpacedRectSide\",\"uuid\":\"81208621-951c-43f9-b655-3502a16ce57a\"},{\"content\":{\"connectorIds\":[\"In4\"],\"side\":\"TOP\"},\"type\":\"ConnectorPlacement.EquallySpacedRectSide\",\"uuid\":\"1012e2be-7d0b-44a9-9a40-bc453950010e\"},{\"content\":{\"connectorIds\":[\"In5\"],\"side\":\"BOTTOM\"},\"type\":\"ConnectorPlacement.EquallySpacedRectSide\",\"uuid\":\"aaef83a2-abb7-4780-82b5-9abad57d39ad\"}]},\"type\":\"ConnectorPlacement.EquallySpacedConnector\",\"uuid\":\"1143871f-aacc-4fa7-a444-9910d5016eff\"}],\"packageUris\":[\"http://schema.mathworks.com/mf0/Connector/R2020b\"],\"version\":\"1.0\"}"
  Sum : Sum  Inputs=|+++
  Sum2 : Sum  Inputs=|+-
  seconds 2 days : Gain  Gain=3600*24
  seconds 2 days1 : Gain  Gain=3600*24*0.001
  time of response : Gain  Gain=1/(30)
  MassFlows : Outport
  wires:
  T/1 -> [T]
  Sum/1 -> [TotalMass]
  [TotalMass] -> Product/2
  Diesel/1 -> Sum/1, Subsystem/1(Diesel)
  seconds 2 days1/1 -> Integrator/1
  Gain/1 -> seconds 2 days1/1
  [a] -> Subsystem/5(a)
  [T] -> Subsystem/4(T)
  time of response/1 -> seconds 2 days/1
  Sum2/1 -> time of response/1
  Product/1 -> Sum2/1  "Target"
  seconds 2 days/1 -> Integrator1/1
  Integrator1/1 -> MassFlows/1, Sum2/2  "previous state"
  Subsystem/1(Out1) -> Product/1  "Target"
  Steam/1 -> Sum/2, Subsystem/2(Steam)
  Air/1 -> Sum/3, Subsystem/3(Air)
  Integrator/1 -> Scope/1, Gain/1, [a]

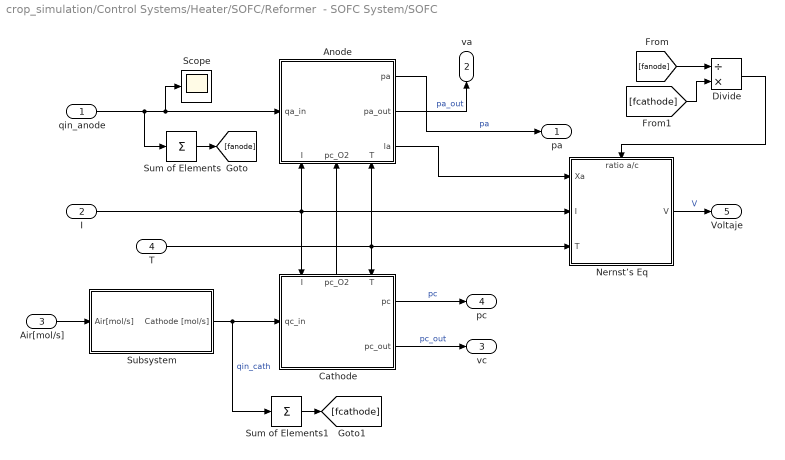
== system crop_simulation/Control Systems/Heater/SOFC/Reformer  - SOFC System/SOFC  ==
  qin_anode : Inport
  I : Inport  Port=2
  Air[mol/s] : Inport  Port=3
  T : Inport  Port=4
  Anode : Subsystem
      settings: PortSchema="{\"entries\":[{\"content\":{\"sides\":[{\"content\":{\"connectorIds\":[\"In1\"]},\"type\":\"ConnectorPlacement.EquallySpacedRectSide\",\"uuid\":\"1d27f661-9cb9-482d-ac43-89e84d52643b\"},{\"content\":{\"connectorIds\":[\"Out1\",\"Out2\",\"Out3\"],\"side\":\"RIGHT\"},\"type\":\"ConnectorPlacement.EquallySpacedRectSide\",\"uuid\":\"62ac897d-5819-4e9c-a19f-e210851aefa2\"},{\"content\":{\"connectorIds\":[],\"side\":\"TOP\"},\"type\":\"ConnectorPlacement.EquallySpacedRectSide\",\"uuid\":\"1380e9d4-c5ac-42ce-b6fc-00336cc8edba\"},{\"content\":{\"connectorIds\":[\"In2\",\"In3\",\"In4\"],\"side\":\"BOTTOM\"},\"type\":\"ConnectorPlacement.EquallySpacedRectSide\",\"uuid\":\"0e36fd1a-38eb-48cb-8834-06d558b43614\"}]},\"type\":\"ConnectorPlacement.EquallySpacedConnector\",\"uuid\":\"79a72313-dbdc-4de5-b88f-787bafe984c7\"}],\"packageUris\":[\"http://schema.mathworks.com/mf0/Connector/R2020b\"],\"version\":\"1.0\"}"
  Cathode : Subsystem
      settings: PortSchema="{\"entries\":[{\"content\":{\"sides\":[{\"content\":{\"connectorIds\":[\"In1\"]},\"type\":\"ConnectorPlacement.EquallySpacedRectSide\",\"uuid\":\"1d27f661-9cb9-482d-ac43-89e84d52643b\"},{\"content\":{\"connectorIds\":[\"Out1\",\"Out2\"],\"side\":\"RIGHT\"},\"type\":\"ConnectorPlacement.EquallySpacedRectSide\",\"uuid\":\"62ac897d-5819-4e9c-a19f-e210851aefa2\"},{\"content\":{\"connectorIds\":[\"In2\",\"Out3\",\"In3\"],\"side\":\"TOP\"},\"type\":\"ConnectorPlacement.EquallySpacedRectSide\",\"uuid\":\"1380e9d4-c5ac-42ce-b6fc-00336cc8edba\"}]},\"type\":\"ConnectorPlacement.EquallySpacedConnector\",\"uuid\":\"79a72313-dbdc-4de5-b88f-787bafe984c7\"}],\"packageUris\":[\"http://schema.mathworks.com/mf0/Connector/R2020b\"],\"version\":\"1.0\"}"
  Divide : Product  Inputs=/*
  "Nernst’s Eq " : Subsystem
      settings: PortSchema="{\"entries\":[{\"content\":{\"sides\":[{\"content\":{\"connectorIds\":[\"In1\",\"In2\",\"In3\"]},\"type\":\"ConnectorPlacement.EquallySpacedRectSide\",\"uuid\":\"1b300774-e64d-4a8a-a2e9-ecdc71723fee\"},{\"content\":{\"connectorIds\":[\"Out1\"],\"side\":\"RIGHT\"},\"type\":\"ConnectorPlacement.EquallySpacedRectSide\",\"uuid\":\"354a04f1-cc66-4a63-8c50-8080316e29e9\"},{\"content\":{\"connectorIds\":[\"In4\"],\"side\":\"TOP\"},\"type\":\"ConnectorPlacement.EquallySpacedRectSide\",\"uuid\":\"b48b7bda-dd37-468f-ab7d-ccd563a69f0b\"}]},\"type\":\"ConnectorPlacement.EquallySpacedConnector\",\"uuid\":\"ddfd4041-6e53-4893-9028-34e5ff9f82d6\"}],\"packageUris\":[\"http://schema.mathworks.com/mf0/Connector/R2020b\"],\"version\":\"1.0\"}"
  Scope : Scope
  Subsystem : Subsystem
  Sum of Elements : Sum  Inputs=+
  Sum of Elements1 : Sum  Inputs=+
  pa : Outport
  va : Outport  Port=2
  vc : Outport  Port=3
  pc : Outport  Port=4
  Voltaje : Outport  Port=5
  wires:
  Air[mol/s]/1 -> Subsystem/1(Air[mol/s])
  Anode/1(pa) -> pa/1  "pa"
  Anode/2(pa_out) -> va/1  "pa_out"
  Cathode/1(pc) -> pc/1  "pc"
  Subsystem/1(Cathode [mol/s]) -> Sum of Elements1/1, Cathode/1(qc_in)  "qin_cath"
  Cathode/3(pc_O2) -> Anode/3(pc_O2)
  Cathode/2(pc_out) -> vc/1  "pc_out"
  I/1 -> Cathode/2(I), "Nernst’s Eq "/2(I), Anode/2(I)
  T/1 -> Cathode/3(T), "Nernst’s Eq "/3(T), Anode/4(T)
  qin_anode/1 -> Scope/1, Anode/1(qa_in), Sum of Elements/1
  "Nernst’s Eq "/1(V) -> Voltaje/1  "V"
  Anode/3(la) -> "Nernst’s Eq "/1(Xa)
  Sum of Elements/1 -> [fanode]
  Sum of Elements1/1 -> [fcathode]
  [fanode] -> Divide/1
  [fcathode] -> Divide/2
  Divide/1 -> "Nernst’s Eq "/4(ratio a/c)

== system crop_simulation/Control Systems/Heater/SOFC/Subsystem2/Continous ==
  Target : Inport
  EPD : Inport  Port=2
  Gain : Gain  Gain=24*3600*0.01
  Integrator : Integrator  InitialCondition=10  LimitOutput=on  UpperSaturationLimit=30  LowerSaturationLimit=1
  Minus : Sum  Inputs=+-
  Scope : Scope  NumInputPorts=2
  Vector Concatenate : Concatenate
  I [A] : Outport
  wires:
  Target/1 -> Minus/1, Vector Concatenate/1
  EPD/1 -> Vector Concatenate/2, Minus/2
  Integrator/1 -> Scope/1, I [A]/1
  Gain/1 -> Integrator/1
  Minus/1 -> Gain/1
  Vector Concatenate/1 -> Scope/2
